simulink library "Absorption_Chiller_ddT"  (Simulink 7.6)
settings: Solver=ode45  StartTime=0.0  StopTime=10.0  RelTol=1e-3
undefined symbols (not defined in the file): A, B, C, Dd
libraries: carnot x5
settings Model: Creator=lena.frank  LastModifiedBy=drhf

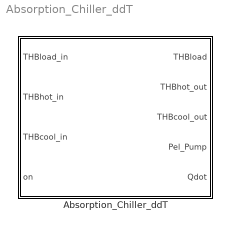
== system Absorption_Chiller_ddT ==
  Absorption_Chiller_ddT : Subsystem  mask(Absorption chiller model){E=1.2, sE=0.42, rE=0.9, sG=0.51, rG=2/0.51, dpe=[100 1e4], dpg=[100 1e4], Pel_p=80}
      mask prompts: E "E (A = 1+E)"; sE "s_e"; rE "r_e"; sG "s_g"; rG "r_g"; dpe "[linear quadratic] massflow dependant pressure drop evaporator in [Pa]"; dpg "[linear quadratic] massflow dependant pressure drop generator in [Pa]"; Pel_p "Pel solution pump [W]"
      mask help:
      | Empirical model of an absorption chiller based on the fitted deltadelta_t'
      | model from A. Kühn (2005) :
      |
      | Linear model:
      |  deltadelta_t'=t_G - A*t_AC + E*t_E
      |  Qdot_E = s_e * deltadelta_t' + r_e
      |  Qdot_G = s_g * deltadelta_t' + r_g
      |
      | Use acm_param.m to determine A, E, s_e, r_e, s_g and r_g with
      | characterisitics of the absorption chiller.
      mask Display: disp('Absorption\nChiller\nDeltaDeltaT\nModel')

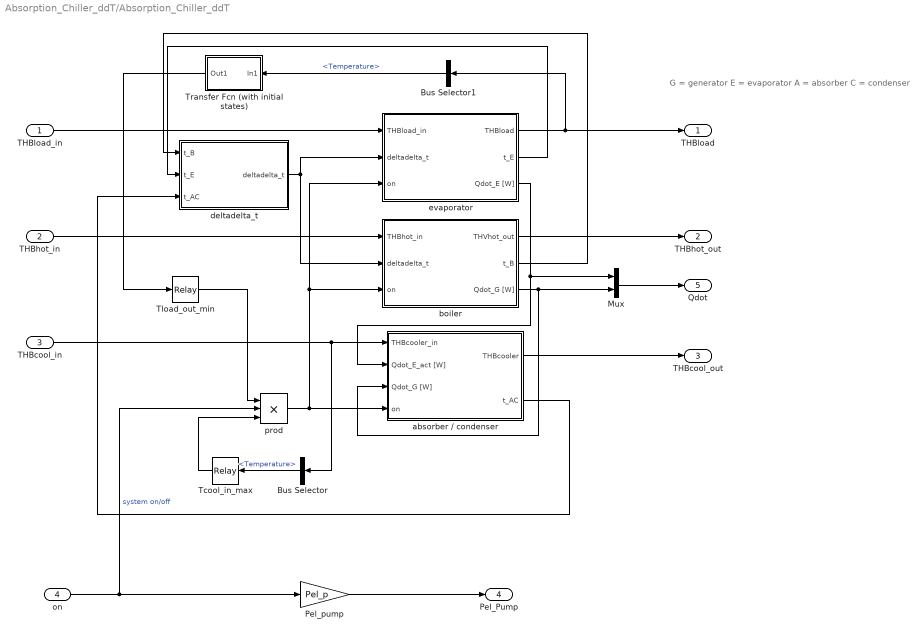
== system Absorption_Chiller_ddT/Absorption_Chiller_ddT ==
  note: G = generator
      | E = evaporator
      | A = absorber
      | C = condenser
  THBload_in : Inport
  THBhot_in : Inport  Port=2
  THBcool_in : Inport  Port=3
  on : Inport  Port=4
  Bus Selector : BusSelector  OutputSignals=Temperature
  Bus Selector1 : BusSelector  OutputSignals=Temperature
  Mux : Mux  Inputs=2
  Pel_pump : Gain  Gain=Pel_p
  Tcool_in_max : Relay  OnSwitchValue=35  OffSwitchValue=30  OnOutputValue=0  OffOutputValue=1
  Tload_out_min : Relay  OnSwitchValue=2  OffSwitchValue=0
  Transfer Fcn (with initial states) : Subsystem  mask(Transfer Function with Initial States){N=[1], D=[10 1], X0=20}
      mask prompts: N "Numerator:"; D "Denominator:"; X0 "Initial conditions:"
      mask help: Vector expressions for numerator, and denominator. Coefficients are in descending powers of s.
      mask init:
      | [A,B,C,Dd]=tf2ss(N,D);if (isempty(X0));[m,n]=size(A);X0=zeros(1,m); end;
      mask Help: Specify the initial states for the transfer function.  The state ordering is determined by the m-file tf2ss.  There is no unique mapping of the states in a transfer function to states in a state-space representation.  However, tf2ss will consistently use the same mapping for a given transfer function.
      mask Display: dpoly(N,D,'s')
  absorber / condenser : Subsystem
  boiler : Subsystem
  deltadelta_t : Subsystem
  evaporator : Subsystem
  prod : Product  Inputs=3
  THBload : Outport
  THBhot_out : Outport  Port=2
  THBcool_out : Outport  Port=3
  Pel_Pump : Outport  Port=4
  Qdot : Outport  Port=5
  wires:
  deltadelta_t/1(deltadelta_t) -> evaporator/2(deltadelta_t), boiler/2(deltadelta_t)
  boiler/3(Qdot_G [W]) -> absorber / condenser/3(Qdot_G [W]), Mux/2
  THBload_in/1 -> evaporator/1(THBload_in)
  boiler/1(THVhot_out) -> THBhot_out/1
  THBhot_in/1 -> boiler/1(THBhot_in)
  THBcool_in/1 -> absorber / condenser/1(THBcooler_in), Bus Selector/1
  absorber / condenser/1(THBcooler) -> THBcool_out/1
  evaporator/1(THBload) -> THBload/1, Bus Selector1/1
  evaporator/2(t_E) -> deltadelta_t/2(t_E)
  evaporator/3(Qdot_E [W]) -> absorber / condenser/2(Qdot_E_act [W]), Mux/1
  boiler/2(t_B) -> deltadelta_t/1(t_B)
  absorber / condenser/2(t_AC) -> deltadelta_t/3(t_AC)
  Pel_pump/1 -> Pel_Pump/1
  Tload_out_min/1 -> prod/1
  prod/1 -> evaporator/3(on), boiler/3(on), absorber / condenser/4(on)
  Bus Selector1/1 -> Transfer Fcn (with initial states)/1(In1)  "<Temperature>"
  Transfer Fcn (with initial states)/1(Out1) -> Tload_out_min/1
  Tcool_in_max/1 -> prod/3
  Bus Selector/1 -> Tcool_in_max/1  "<Temperature>"
  on/1 -> Pel_pump/1, prod/2  "system on/off"
  Mux/1 -> Qdot/1

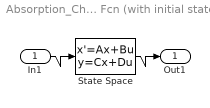
== system Absorption_Chiller_ddT/Absorption_Chiller_ddT/Transfer Fcn (with initial states) ==
  In1 : Inport
  State Space : StateSpace  A=A  B=B  C=C  D=Dd  X0=X0
  Out1 : Outport  InitialOutput=0
  wires:
  State Space/1 -> Out1/1
  In1/1 -> State Space/1

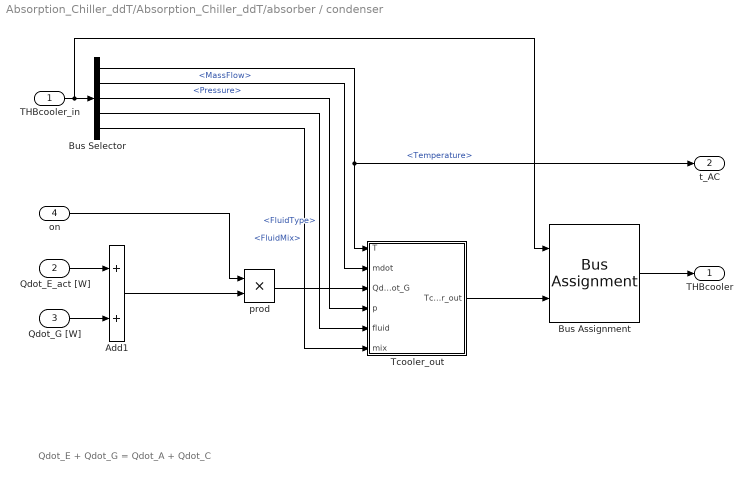
== system Absorption_Chiller_ddT/Absorption_Chiller_ddT/absorber / condenser ==
  note: Qdot_E + Qdot_G = Qdot_A + Qdot_C
  THBcooler_in : Inport
  Qdot_E_act [W] : Inport  Port=2
  Qdot_G [W] : Inport  Port=3
  on : Inport  Port=4
  Add1 : Sum
  Bus Assignment : BusAssignment  AssignedSignals=Temperature
  Bus Selector : BusSelector  OutputSignals=Temperature,MassFlow,Pressure,FluidType,FluidMix
  Tcooler_out : Subsystem
  prod : Product
  THBcooler : Outport
  t_AC : Outport  Port=2
  wires:
  Bus Selector/2 -> Tcooler_out/2(mdot)  "<MassFlow>"
  Bus Selector/1 -> Tcooler_out/1(T), t_AC/1  "<Temperature>"
  Bus Selector/3 -> Tcooler_out/4(p)  "<Pressure>"
  Bus Selector/4 -> Tcooler_out/5(fluid)  "<FluidType>"
  Bus Selector/5 -> Tcooler_out/6(mix)  "<FluidMix>"
  THBcooler_in/1 -> Bus Selector/1, Bus Assignment/1
  Qdot_E_act [W]/1 -> Add1/1
  Qdot_G [W]/1 -> Add1/2
  on/1 -> prod/1
  Add1/1 -> prod/2
  prod/1 -> Tcooler_out/3(Qdot_E + Qdot_G)
  Bus Assignment/1 -> THBcooler/1
  Tcooler_out/1(Tcooler_out) -> Bus Assignment/2

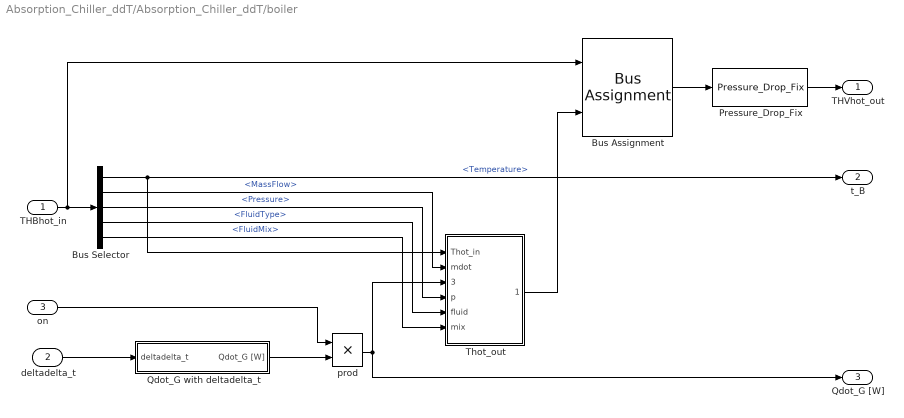
== system Absorption_Chiller_ddT/Absorption_Chiller_ddT/boiler ==
  THBhot_in : Inport
  deltadelta_t : Inport  Port=2
  on : Inport  Port=3
  Bus Assignment : BusAssignment  AssignedSignals=Temperature
  Bus Selector : BusSelector  OutputSignals=Temperature,MassFlow,Pressure,FluidType,FluidMix
  Pressure_Drop_Fix : carnot/Basic/Pressure_Drop/Pressure_Drop_Fix  SystemSampleTime=-1  con=0  lin=dpg(1)  qua=dpg(2)
  Qdot_G with deltadelta_t : Subsystem
  Thot_out : Subsystem
  prod : Product
  THVhot_out : Outport
  t_B : Outport  Port=2
  Qdot_G [W] : Outport  Port=3
  wires:
  Bus Selector/2 -> Thot_out/2(mdot)  "<MassFlow>"
  Bus Selector/1 -> Thot_out/1(Thot_in), t_B/1  "<Temperature>"
  Bus Selector/3 -> Thot_out/4(p)  "<Pressure>"
  Bus Selector/4 -> Thot_out/5(fluid)  "<FluidType>"
  Bus Selector/5 -> Thot_out/6(mix)  "<FluidMix>"
  deltadelta_t/1 -> Qdot_G with deltadelta_t/1(deltadelta_t)
  prod/1 -> Thot_out/3(Qdot_G), Qdot_G [W]/1
  on/1 -> prod/1
  Qdot_G with deltadelta_t/1(Qdot_G [W]) -> prod/2
  THBhot_in/1 -> Bus Selector/1, Bus Assignment/1
  Bus Assignment/1 -> Pressure_Drop_Fix/1
  Thot_out/1(Thot_out) -> Bus Assignment/2
  Pressure_Drop_Fix/1 -> THVhot_out/1

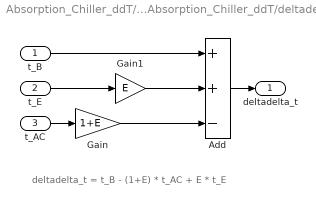
== system Absorption_Chiller_ddT/Absorption_Chiller_ddT/deltadelta_t ==
  note: deltadelta_t = t_B - (1+E) * t_AC + E * t_E
  t_B : Inport
  t_E : Inport  Port=2
  t_AC : Inport  Port=3
  Add : Sum  Inputs=++-
  Gain : Gain  Gain=1+E
  Gain1 : Gain  Gain=E
  deltadelta_t : Outport
  wires:
  Gain/1 -> Add/3
  Gain1/1 -> Add/2
  t_B/1 -> Add/1
  Add/1 -> deltadelta_t/1
  t_E/1 -> Gain1/1
  t_AC/1 -> Gain/1

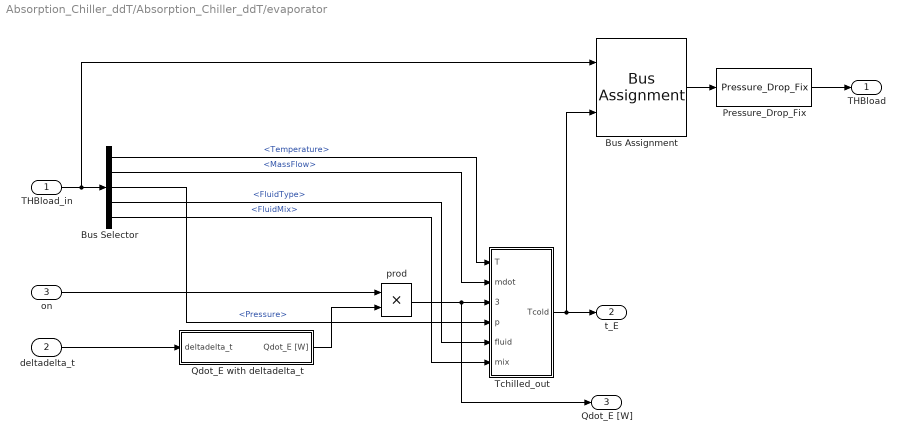
== system Absorption_Chiller_ddT/Absorption_Chiller_ddT/evaporator ==
  THBload_in : Inport
  deltadelta_t : Inport  Port=2
  on : Inport  Port=3
  Bus Assignment : BusAssignment  AssignedSignals=Temperature
  Bus Selector : BusSelector  OutputSignals=Temperature,MassFlow,Pressure,FluidType,FluidMix
  Pressure_Drop_Fix : carnot/Basic/Pressure_Drop/Pressure_Drop_Fix  SystemSampleTime=-1  con=0  lin=dpe(1)  qua=dpe(2)
  Qdot_E with deltadelta_t : Subsystem
  Tchilled_out : Subsystem
  prod : Product
  THBload : Outport
  t_E : Outport  Port=2
  Qdot_E [W] : Outport  Port=3
  wires:
  Bus Selector/2 -> Tchilled_out/2(mdot)  "<MassFlow>"
  Bus Selector/1 -> Tchilled_out/1(T)  "<Temperature>"
  Bus Selector/4 -> Tchilled_out/5(fluid)  "<FluidType>"
  Bus Selector/5 -> Tchilled_out/6(mix)  "<FluidMix>"
  deltadelta_t/1 -> Qdot_E with deltadelta_t/1(deltadelta_t)
  Tchilled_out/1(Tcold) -> t_E/1, Bus Assignment/2
  Bus Selector/3 -> Tchilled_out/4(p)  "<Pressure>"
  on/1 -> prod/1
  prod/1 -> Tchilled_out/3(Qdot_E), Qdot_E [W]/1
  Qdot_E with deltadelta_t/1(Qdot_E [W]) -> prod/2
  THBload_in/1 -> Bus Selector/1, Bus Assignment/1
  Bus Assignment/1 -> Pressure_Drop_Fix/1
  Pressure_Drop_Fix/1 -> THBload/1

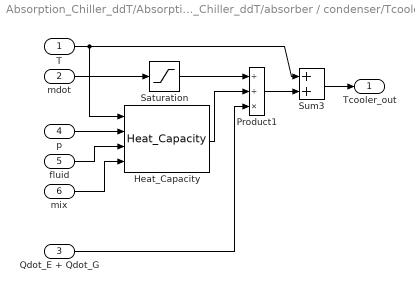
== system Absorption_Chiller_ddT/Absorption_Chiller_ddT/absorber / condenser/Tcooler_out ==
  T : Inport
  mdot : Inport  Port=2
  Qdot_E + Qdot_G : Inport  Port=3
  p : Inport  Port=4
  fluid : Inport  Port=5
  mix : Inport  Port=6
  Heat_Capacity : carnot/Basic/Material_Properties/Heat_Capacity  SystemSampleTime=-1  VariantObject=CarlibClassic  INPUTARGUMENTS=state variables (classic)  DEBUGLEVEL=DEBUGLEVEL  MAXTOTALWARNINGS=inf  MAXCONSECUTIVEWARNINGS=inf  WRITETOFILE=0  FILENAME='errors.txt'
  Product1 : Product  Inputs=//*  SaturateOnIntegerOverflow=on  InputSameDT=on  OutDataTypeStr=Inherit: Same as first input
  Saturation : Saturate  UpperLimit=inf  LowerLimit=1e-5
  Sum3 : Sum  SaturateOnIntegerOverflow=on  InputSameDT=on  OutDataTypeStr=Inherit: Same as first input
  Tcooler_out : Outport  InitialOutput=0
  wires:
  mix/1 -> Heat_Capacity/4
  fluid/1 -> Heat_Capacity/3
  p/1 -> Heat_Capacity/2
  T/1 -> Sum3/1, Heat_Capacity/1
  Heat_Capacity/1 -> Product1/2
  Product1/1 -> Sum3/2
  mdot/1 -> Saturation/1
  Sum3/1 -> Tcooler_out/1
  Saturation/1 -> Product1/1
  Qdot_E + Qdot_G/1 -> Product1/3

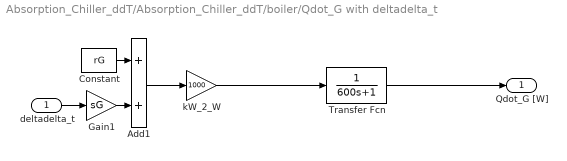
== system Absorption_Chiller_ddT/Absorption_Chiller_ddT/boiler/Qdot_G with deltadelta_t ==
  deltadelta_t : Inport
  Add1 : Sum
  Constant : Constant  Value=rG
  Gain1 : Gain  Gain=sG
  Transfer Fcn : TransferFcn  Denominator=[600 1]
  kW_2_W : Gain  Gain=1000
  Qdot_G [W] : Outport
  wires:
  Constant/1 -> Add1/1
  Gain1/1 -> Add1/2
  deltadelta_t/1 -> Gain1/1
  Add1/1 -> kW_2_W/1
  kW_2_W/1 -> Transfer Fcn/1
  Transfer Fcn/1 -> Qdot_G [W]/1

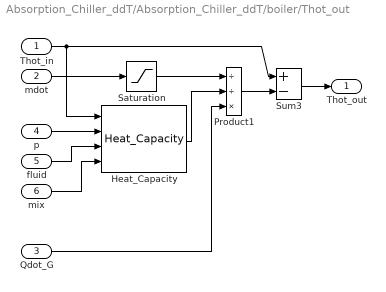
== system Absorption_Chiller_ddT/Absorption_Chiller_ddT/boiler/Thot_out ==
  Thot_in : Inport
  mdot : Inport  Port=2
  Qdot_G : Inport  Port=3
  p : Inport  Port=4
  fluid : Inport  Port=5
  mix : Inport  Port=6
  Heat_Capacity : carnot/Basic/Material_Properties/Heat_Capacity  SystemSampleTime=-1  VariantObject=CarlibClassic  INPUTARGUMENTS=state variables (classic)  DEBUGLEVEL=DEBUGLEVEL  MAXTOTALWARNINGS=inf  MAXCONSECUTIVEWARNINGS=inf  WRITETOFILE=0  FILENAME='errors.txt'
  Product1 : Product  Inputs=//*  SaturateOnIntegerOverflow=on  InputSameDT=on  OutDataTypeStr=Inherit: Same as first input
  Saturation : Saturate  UpperLimit=inf  LowerLimit=1e-5
  Sum3 : Sum  Inputs=+-  SaturateOnIntegerOverflow=on  InputSameDT=on  OutDataTypeStr=Inherit: Same as first input
  Thot_out : Outport  InitialOutput=0
  wires:
  mix/1 -> Heat_Capacity/4
  fluid/1 -> Heat_Capacity/3
  p/1 -> Heat_Capacity/2
  Thot_in/1 -> Sum3/1, Heat_Capacity/1
  Heat_Capacity/1 -> Product1/2
  Product1/1 -> Sum3/2
  mdot/1 -> Saturation/1
  Sum3/1 -> Thot_out/1
  Saturation/1 -> Product1/1
  Qdot_G/1 -> Product1/3

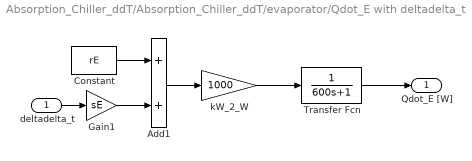
== system Absorption_Chiller_ddT/Absorption_Chiller_ddT/evaporator/Qdot_E with deltadelta_t ==
  deltadelta_t : Inport
  Add1 : Sum
  Constant : Constant  Value=rE
  Gain1 : Gain  Gain=sE
  Transfer Fcn : TransferFcn  Denominator=[600 1]
  kW_2_W : Gain  Gain=1000
  Qdot_E [W] : Outport
  wires:
  Constant/1 -> Add1/1
  Gain1/1 -> Add1/2
  deltadelta_t/1 -> Gain1/1
  Add1/1 -> kW_2_W/1
  kW_2_W/1 -> Transfer Fcn/1
  Transfer Fcn/1 -> Qdot_E [W]/1

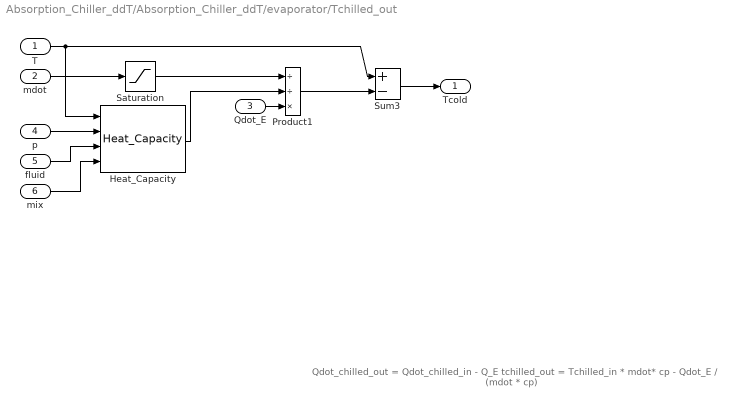
== system Absorption_Chiller_ddT/Absorption_Chiller_ddT/evaporator/Tchilled_out ==
  note: Qdot_chilled_out = Qdot_chilled_in - Q_E
      | tchilled_out = Tchilled_in * mdot* cp - Qdot_E / (mdot * cp)
  T : Inport
  mdot : Inport  Port=2
  Qdot_E : Inport  Port=3
  p : Inport  Port=4
  fluid : Inport  Port=5
  mix : Inport  Port=6
  Heat_Capacity : carnot/Basic/Material_Properties/Heat_Capacity  SystemSampleTime=-1  VariantObject=CarlibClassic  INPUTARGUMENTS=state variables (classic)  DEBUGLEVEL=DEBUGLEVEL  MAXTOTALWARNINGS=inf  MAXCONSECUTIVEWARNINGS=inf  WRITETOFILE=0  FILENAME='errors.txt'
  Product1 : Product  Inputs=//*  SaturateOnIntegerOverflow=on  InputSameDT=on  OutDataTypeStr=Inherit: Same as first input
  Saturation : Saturate  UpperLimit=inf  LowerLimit=1e-5
  Sum3 : Sum  Inputs=+-  SaturateOnIntegerOverflow=on  InputSameDT=on  OutDataTypeStr=Inherit: Same as first input
  Tcold : Outport  InitialOutput=0
  wires:
  mix/1 -> Heat_Capacity/4
  fluid/1 -> Heat_Capacity/3
  p/1 -> Heat_Capacity/2
  T/1 -> Sum3/1, Heat_Capacity/1
  Heat_Capacity/1 -> Product1/2
  Sum3/1 -> Tcold/1
  Saturation/1 -> Product1/1
  mdot/1 -> Saturation/1
  Qdot_E/1 -> Product1/3
  Product1/1 -> Sum3/2
